simulink model "Speedmeter_harness"  (R2019b)
settings: Solver=FixedStepDiscrete  StartTime=0  StopTime=0.58999999999999997  FixedStep=0.01  RelTol=1e-3
undefined symbols (not defined in the file): Const16_0, Const16_2, Const16_210, Const16_340, Const16_350, Const16_4, Const8_0, Const8_1, Const8_2, Const8_4, ConstFL_00879, ConstFL_01, ConstFL_03516, ConstFL_1_6093, sigbuilder_block, STEP_TIME
libraries: simulink x2
(part 2 of 2)

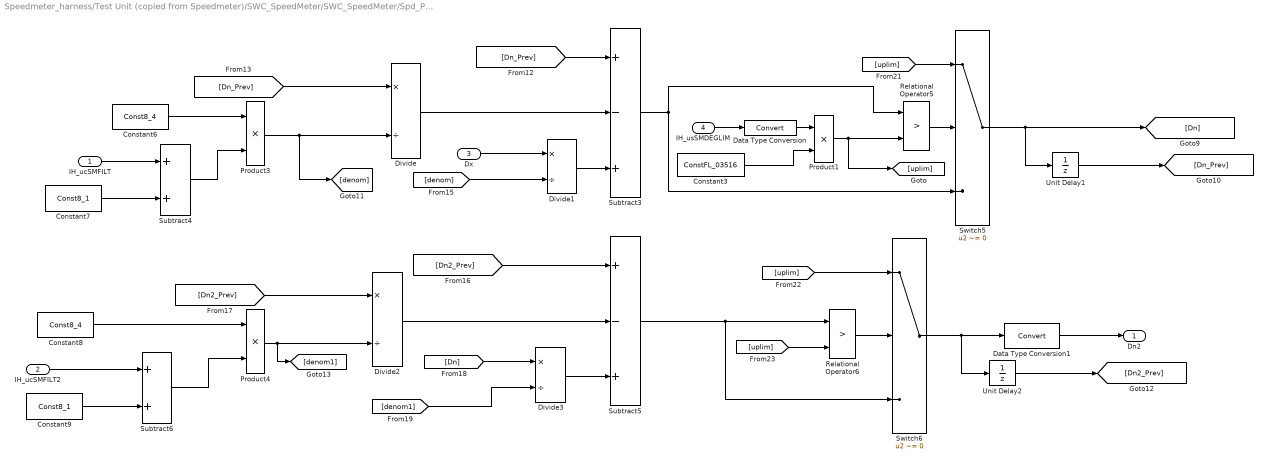
== system Speedmeter_harness/Test Unit (copied from Speedmeter)/SWC_SpeedMeter/SWC_SpeedMeter/Spd_Pointer/Filter ==
  IH_ucSMFILT : Inport  OutMin=0  OutMax=7  OutDataTypeStr=fixdt(0,8,1,0)  SampleTime=STEP_TIME
  IH_ucSMFILT2 : Inport  Port=2  OutMin=0  OutMax=7  OutDataTypeStr=fixdt(0,8,1,0)  SampleTime=STEP_TIME
  Dx : Inport  Port=3  SampleTime=STEP_TIME
  IH_usSMDEGLIM : Inport  Port=4  OutMin=0  OutMax=1023  SampleTime=STEP_TIME
  Constant3 : Constant  Value=ConstFL_03516  OutDataTypeStr=fixdt(0,32,0.0001,0)  SampleTime=STEP_TIME
  Constant6 : Constant  Value=Const8_4  SampleTime=STEP_TIME
  Constant7 : Constant  Value=Const8_1  OutDataTypeStr=uint8  SampleTime=STEP_TIME
  Constant8 : Constant  Value=Const8_4  SampleTime=STEP_TIME
  Constant9 : Constant  Value=Const8_1  SampleTime=STEP_TIME
  Data Type Conversion : DataTypeConversion
  Data Type Conversion1 : DataTypeConversion  SaturateOnIntegerOverflow=on
  Divide{,1..3} (4 alike) : Product  Inputs=*/  OutDataTypeStr=Inherit: Inherit via back propagation  InputSameDT=on
  Product1 : Product  OutDataTypeStr=fixdt(1,32,0.0001,0)  InputSameDT=on
  Product3 : Product  OutDataTypeStr=fixdt(1,32,0.0001,0)  InputSameDT=on
  Product4 : Product  OutDataTypeStr=fixdt(1,32,0.0001,0)  InputSameDT=on
  Relational Operator5 : RelationalOperator  Operator=>  OutDataTypeStr=boolean  RndMeth=Simplest  InputSameDT=on
  Relational Operator6 : RelationalOperator  Operator=>  OutDataTypeStr=boolean  RndMeth=Simplest  InputSameDT=on
  Subtract3 : Sum  Inputs=+-+  InputSameDT=on
  Subtract4 : Sum  InputSameDT=on
  Subtract5 : Sum  Inputs=+-+  OutDataTypeStr=Inherit: Inherit via back propagation  InputSameDT=on
  Subtract6 : Sum  InputSameDT=on
  Switch5 : Switch  Criteria=u2 ~= 0  InputSameDT=on
  Switch6 : Switch  Criteria=u2 ~= 0  OutDataTypeStr=Inherit: Inherit via back propagation  InputSameDT=on
  Unit Delay1 : UnitDelay  SampleTime=-1  HasFrameUpgradeWarning=on
  Unit Delay2 : UnitDelay  SampleTime=-1  HasFrameUpgradeWarning=on
  Dn2 : Outport  SampleTime=STEP_TIME  VectorParamsAs1DForOutWhenUnconnected=off
  wires:
  Divide1/1 -> Subtract3/3
  IH_ucSMFILT/1 -> Subtract4/1
  Subtract5/1 -> Switch6/3, Relational Operator6/1
  Constant9/1 -> Subtract6/2
  Subtract6/1 -> Product4/2
  [uplim] -> Switch5/1
  Divide3/1 -> Subtract5/3
  Switch6/1 -> Unit Delay2/1, Data Type Conversion1/1
  [Dn2_Prev] -> Divide2/1
  [Dn_Prev] -> Divide/1
  Unit Delay2/1 -> [Dn2_Prev]
  [uplim] -> Switch6/1
  [denom] -> Divide1/2
  Divide/1 -> Subtract3/2
  Data Type Conversion/1 -> Product1/1
  [Dn_Prev] -> Subtract3/1
  Relational Operator6/1 -> Switch6/2
  Constant7/1 -> Subtract4/2
  IH_usSMDEGLIM/1 -> Data Type Conversion/1
  Relational Operator5/1 -> Switch5/2
  Dx/1 -> Divide1/1
  Constant3/1 -> Product1/2
  IH_ucSMFILT2/1 -> Subtract6/1
  Constant8/1 -> Product4/1
  [denom1] -> Divide3/2
  [Dn] -> Divide3/1
  Product4/1 -> Divide2/2, [denom1]
  Product1/1 -> Relational Operator5/2, [uplim]
  Unit Delay1/1 -> [Dn_Prev]
  Switch5/1 -> [Dn], Unit Delay1/1
  Product3/1 -> [denom], Divide/2
  Subtract3/1 -> Switch5/3, Relational Operator5/1
  Subtract4/1 -> Product3/2
  [Dn2_Prev] -> Subtract5/1
  [uplim] -> Relational Operator6/2
  Constant6/1 -> Product3/1
  Divide2/1 -> Subtract5/2
  Data Type Conversion1/1 -> Dn2/1

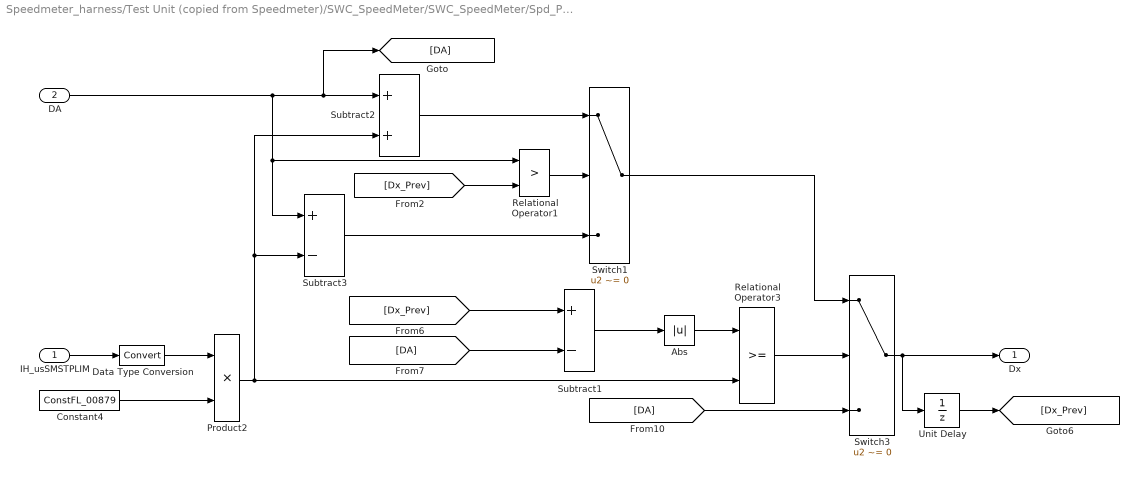
== system Speedmeter_harness/Test Unit (copied from Speedmeter)/SWC_SpeedMeter/SWC_SpeedMeter/Spd_Pointer/InputLimitProccess ==
  IH_usSMSTPLIM : Inport  SampleTime=STEP_TIME
  DA : Inport  Port=2  SampleTime=STEP_TIME
  Abs : Abs  OutDataTypeStr=fixdt(1,32,0.0001,0)
  Constant4 : Constant  Value=ConstFL_00879  OutDataTypeStr=fixdt(0,32,0.0001,0)  SampleTime=STEP_TIME
  Data Type Conversion : DataTypeConversion
  Product2 : Product  OutDataTypeStr=Inherit: Inherit via back propagation  InputSameDT=on
  Relational Operator1 : RelationalOperator  Operator=>  OutDataTypeStr=boolean  RndMeth=Simplest  InputSameDT=on
  Relational Operator3 : RelationalOperator  OutDataTypeStr=boolean  RndMeth=Simplest  InputSameDT=on
  Subtract1 : Sum  Inputs=+-  InputSameDT=on
  Subtract2 : Sum  InputSameDT=on
  Subtract3 : Sum  Inputs=+-  InputSameDT=on
  Switch1 : Switch  Criteria=u2 ~= 0  OutDataTypeStr=Inherit: Inherit via back propagation  InputSameDT=on
  Switch3 : Switch  Criteria=u2 ~= 0  OutDataTypeStr=Inherit: Inherit via back propagation  InputSameDT=on
  Unit Delay : UnitDelay  SampleTime=-1  HasFrameUpgradeWarning=on
  Dx : Outport  SampleTime=STEP_TIME  VectorParamsAs1DForOutWhenUnconnected=off
  wires:
  Unit Delay/1 -> [Dx_Prev]
  DA/1 -> Subtract2/1, [DA], Relational Operator1/1, Subtract3/1
  [Dx_Prev] -> Subtract1/1
  Product2/1 -> Subtract3/2, Subtract2/2, Relational Operator3/2
  Data Type Conversion/1 -> Product2/1
  IH_usSMSTPLIM/1 -> Data Type Conversion/1
  Abs/1 -> Relational Operator3/1
  [DA] -> Switch3/3
  Switch3/1 -> Unit Delay/1, Dx/1
  Subtract1/1 -> Abs/1
  Subtract2/1 -> Switch1/1
  [DA] -> Subtract1/2
  Relational Operator3/1 -> Switch3/2
  Relational Operator1/1 -> Switch1/2
  Switch1/1 -> Switch3/1
  Subtract3/1 -> Switch1/3
  [Dx_Prev] -> Relational Operator1/2
  Constant4/1 -> Product2/2

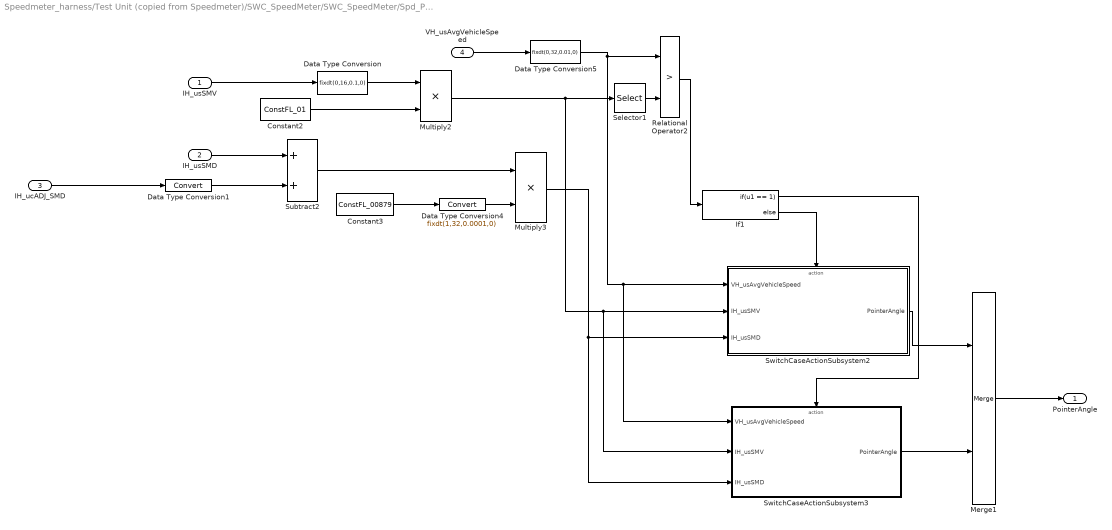
== system Speedmeter_harness/Test Unit (copied from Speedmeter)/SWC_SpeedMeter/SWC_SpeedMeter/Spd_Pointer/PointerAngleCalculation ==
  IH_usSMV : Inport  SampleTime=STEP_TIME
  IH_usSMD : Inport  Port=2  SampleTime=STEP_TIME
  IH_ucADJ_SMD : Inport  Port=3  SampleTime=STEP_TIME
  VH_usAvgVehicleSpeed : Inport  Port=4  SampleTime=STEP_TIME
  Constant2 : Constant  Value=ConstFL_01  SampleTime=STEP_TIME
  Constant3 : Constant  Value=ConstFL_00879  SampleTime=STEP_TIME
  Data Type Conversion : DataTypeConversion  OutDataTypeStr=fixdt(0,16,0.1,0)
  Data Type Conversion1 : DataTypeConversion
  Data Type Conversion4 : DataTypeConversion  OutDataTypeStr=fixdt(1,32,0.0001,0)
  Data Type Conversion5 : DataTypeConversion  OutDataTypeStr=fixdt(0,32,0.01,0)
  If1 : If  IfExpression=u1 == 1
  Merge1 : Merge  InitialOutput=0
  Multiply2 : Product  OutDataTypeStr=fixdt(0,32,0.01,0)  InputSameDT=on
  Multiply3 : Product  InputSameDT=on  OutDataTypeStr=Inherit: Same as first input
  Relational Operator2 : RelationalOperator  Operator=>  OutDataTypeStr=boolean  RndMeth=Simplest
  Selector1 : Selector  IndexMode=Zero-based  InputPortWidth=13  IndexOptions=Index vector (dialog)  Indices=[12]  OutputSizes=1
  Subtract2 : Sum  OutDataTypeStr=Inherit: Inherit via back propagation  InputSameDT=on
  SwitchCaseActionSubsystem2 : Subsystem  TreatAsAtomicUnit=on
  SwitchCaseActionSubsystem3 : Subsystem  TreatAsAtomicUnit=on
  PointerAngle : Outport  SampleTime=STEP_TIME  VectorParamsAs1DForOutWhenUnconnected=off
  wires:
  Data Type Conversion1/1 -> Subtract2/2
  Multiply3/1 -> SwitchCaseActionSubsystem3/3(IH_usSMD), SwitchCaseActionSubsystem2/3(IH_usSMD)
  IH_usSMV/1 -> Data Type Conversion/1
  VH_usAvgVehicleSpeed/1 -> Data Type Conversion5/1
  Constant3/1 -> Data Type Conversion4/1
  SwitchCaseActionSubsystem2/1(PointerAngle) -> Merge1/1
  Data Type Conversion/1 -> Multiply2/1
  Data Type Conversion5/1 -> Relational Operator2/1, SwitchCaseActionSubsystem3/1(VH_usAvgVehicleSpeed), SwitchCaseActionSubsystem2/1(VH_usAvgVehicleSpeed)
  Subtract2/1 -> Multiply3/1
  Relational Operator2/1 -> If1/1
  Merge1/1 -> PointerAngle/1
  Multiply2/1 -> SwitchCaseActionSubsystem3/2(IH_usSMV), SwitchCaseActionSubsystem2/2(IH_usSMV), Selector1/1
  Data Type Conversion4/1 -> Multiply3/2
  SwitchCaseActionSubsystem3/1(PointerAngle) -> Merge1/2
  If1/2 -> SwitchCaseActionSubsystem2/Action
  IH_usSMD/1 -> Subtract2/1
  If1/1 -> SwitchCaseActionSubsystem3/Action
  IH_ucADJ_SMD/1 -> Data Type Conversion1/1
  Selector1/1 -> Relational Operator2/2
  Constant2/1 -> Multiply2/2

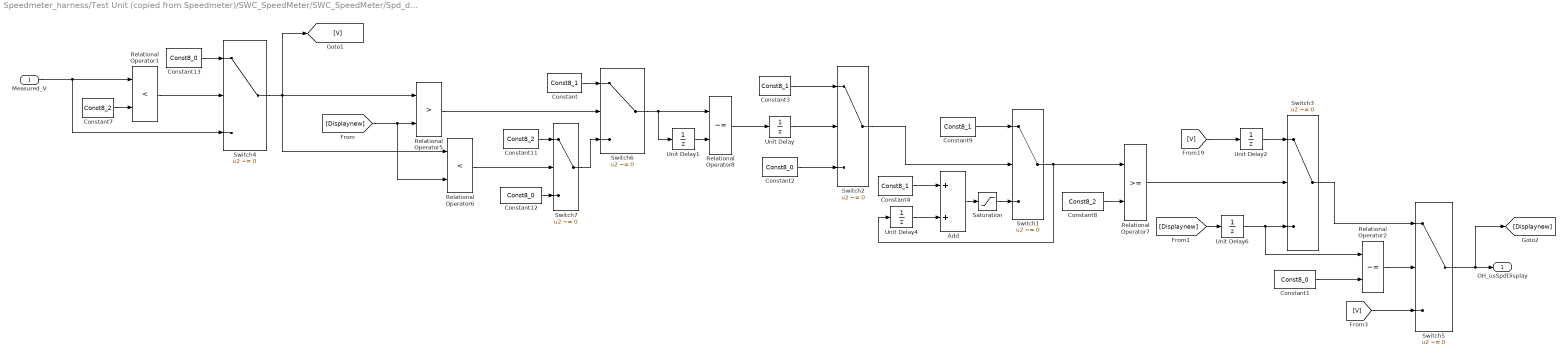
== system Speedmeter_harness/Test Unit (copied from Speedmeter)/SWC_SpeedMeter/SWC_SpeedMeter/Spd_disp/Displayfilter ==
  Measured_V : Inport  OutDataTypeStr=fixdt(0,16,1,0)
  Add : Sum  InputSameDT=on
  Constant{,3..4,9} (4 alike) : Constant  Value=Const8_1
  Constant1 : Constant  Value=Const8_0  OutDataTypeStr=Inherit: Inherit via back propagation
  Constant11 : Constant  Value=Const8_2
  Constant12 : Constant  Value=Const8_0
  Constant13 : Constant  Value=Const8_0  OutDataTypeStr=Inherit: Inherit via back propagation
  Constant2 : Constant  Value=Const8_0
  Constant7 : Constant  Value=Const8_2  OutDataTypeStr=Inherit: Inherit via back propagation
  Constant8 : Constant  Value=Const8_2
  Relational Operator1 : RelationalOperator  Operator=<  OutDataTypeStr=boolean  RndMeth=Simplest  InputSameDT=on
  Relational Operator2 : RelationalOperator  Operator=~=  OutDataTypeStr=boolean  RndMeth=Simplest  InputSameDT=on
  Relational Operator5 : RelationalOperator  Operator=>  OutDataTypeStr=boolean  RndMeth=Simplest  InputSameDT=on
  Relational Operator6 : RelationalOperator  Operator=<  OutDataTypeStr=boolean  RndMeth=Simplest  InputSameDT=on
  Relational Operator7 : RelationalOperator  OutDataTypeStr=boolean  RndMeth=Simplest  InputSameDT=on
  Relational Operator8 : RelationalOperator  Operator=~=  OutDataTypeStr=boolean  RndMeth=Simplest  InputSameDT=on
  Saturation : Saturate  UpperLimit=3  LowerLimit=1  OutDataTypeStr=uint8
  Switch1 : Switch  Criteria=u2 ~= 0  Threshold=2  InputSameDT=on
  Switch2 : Switch  Criteria=u2 ~= 0  Threshold=2  InputSameDT=on
  Switch3 : Switch  Criteria=u2 ~= 0  OutDataTypeStr=Inherit: Inherit via back propagation  InputSameDT=on
  Switch{4..7} (4 alike) : Switch  Criteria=u2 ~= 0  InputSameDT=on
  Unit Delay{,1..2,4,6} (5 alike) : UnitDelay  SampleTime=-1  HasFrameUpgradeWarning=on
  OH_usSpdDisplay : Outport  OutDataTypeStr=fixdt(0,16,1,0)  VectorParamsAs1DForOutWhenUnconnected=off
  wires:
  Switch2/1 -> Switch1/2
  Switch5/1 -> OH_usSpdDisplay/1, [Displaynew]
  Relational Operator8/1 -> Unit Delay/1
  Unit Delay4/1 -> Add/2
  Relational Operator2/1 -> Switch5/2
  Switch4/1 -> Relational Operator6/1, Relational Operator5/1, [V]
  Constant8/1 -> Relational Operator7/2
  [Displaynew] -> Relational Operator6/2, Relational Operator5/2
  Switch1/1 -> Unit Delay4/1, Relational Operator7/1
  Relational Operator1/1 -> Switch4/2
  Unit Delay6/1 -> Switch3/3, Relational Operator2/1
  Constant4/1 -> Add/1
  Unit Delay1/1 -> Relational Operator8/2
  Switch6/1 -> Relational Operator8/1, Unit Delay1/1
  Constant2/1 -> Switch2/3
  Add/1 -> Saturation/1
  Unit Delay/1 -> Switch2/2
  Switch3/1 -> Switch5/1
  Constant11/1 -> Switch7/1
  Constant3/1 -> Switch2/1
  Measured_V/1 -> Relational Operator1/1, Switch4/3
  Constant12/1 -> Switch7/3
  [Displaynew] -> Unit Delay6/1
  Constant/1 -> Switch6/1
  Switch7/1 -> Switch6/3
  Constant9/1 -> Switch1/1
  Constant7/1 -> Relational Operator1/2
  Saturation/1 -> Switch1/3
  Unit Delay2/1 -> Switch3/1
  Constant1/1 -> Relational Operator2/2
  [V] -> Switch5/3
  Relational Operator5/1 -> Switch6/2
  Relational Operator6/1 -> Switch7/2
  Relational Operator7/1 -> Switch3/2
  Constant13/1 -> Switch4/1
  [V] -> Unit Delay2/1

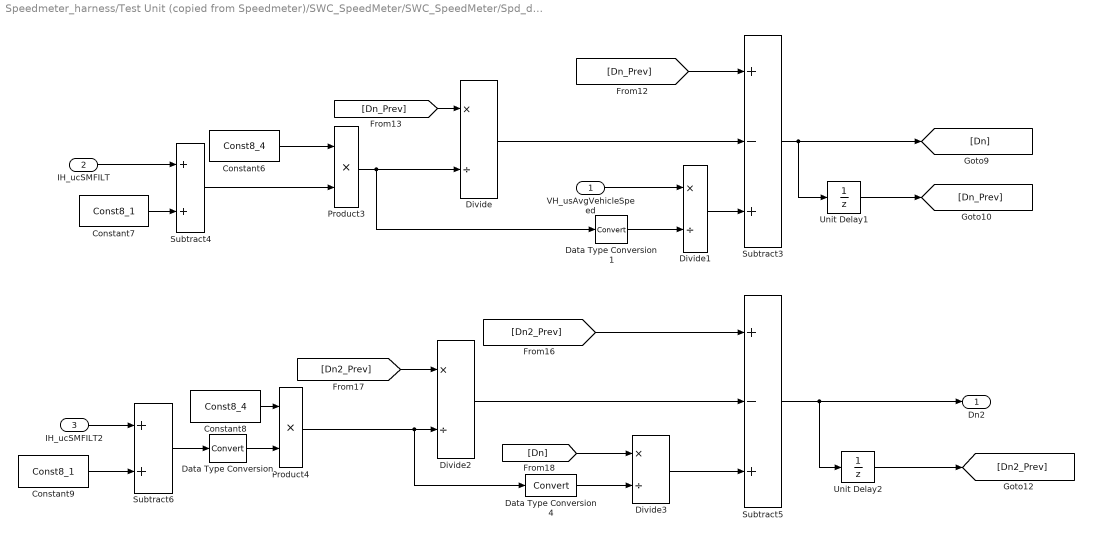
== system Speedmeter_harness/Test Unit (copied from Speedmeter)/SWC_SpeedMeter/SWC_SpeedMeter/Spd_disp/FilteringProcess ==
  VH_usAvgVehicleSpeed : Inport  SampleTime=STEP_TIME
  IH_ucSMFILT : Inport  Port=2  OutDataTypeStr=fixdt(0,8,1,0)  SampleTime=STEP_TIME
  IH_ucSMFILT2 : Inport  Port=3  OutDataTypeStr=fixdt(0,8,1,0)  SampleTime=STEP_TIME
  Constant6 : Constant  Value=Const8_4  SampleTime=STEP_TIME
  Constant7 : Constant  Value=Const8_1  SampleTime=STEP_TIME
  Constant8 : Constant  Value=Const8_4  SampleTime=STEP_TIME
  Constant9 : Constant  Value=Const8_1  SampleTime=STEP_TIME
  Data Type Conversion : DataTypeConversion
  Data Type Conversion1 : DataTypeConversion
  Data Type Conversion4 : DataTypeConversion
  Divide{,1..3} (4 alike) : Product  Inputs=*/  OutDataTypeStr=fixdt(0,16,0.1,0)  InputSameDT=on
  Product3 : Product  OutDataTypeStr=Inherit: Inherit via back propagation  InputSameDT=on
  Product4 : Product  OutDataTypeStr=Inherit: Inherit via back propagation  InputSameDT=on
  Subtract3 : Sum  Inputs=+-+  InputSameDT=on
  Subtract4 : Sum  InputSameDT=on
  Subtract5 : Sum  Inputs=+-+  InputSameDT=on
  Subtract6 : Sum  OutDataTypeStr=uint16  InputSameDT=on
  Unit Delay1 : UnitDelay  SampleTime=-1  HasFrameUpgradeWarning=on
  Unit Delay2 : UnitDelay  SampleTime=-1  HasFrameUpgradeWarning=on
  Dn2 : Outport  SampleTime=STEP_TIME  VectorParamsAs1DForOutWhenUnconnected=off
  wires:
  Unit Delay2/1 -> [Dn2_Prev]
  [Dn2_Prev] -> Subtract5/1
  Data Type Conversion4/1 -> Divide3/2
  Unit Delay1/1 -> [Dn_Prev]
  [Dn_Prev] -> Subtract3/1
  Data Type Conversion1/1 -> Divide1/2
  Data Type Conversion/1 -> Product4/2
  Constant9/1 -> Subtract6/2
  Divide1/1 -> Subtract3/3
  Constant8/1 -> Product4/1
  Divide/1 -> Subtract3/2
  Subtract3/1 -> [Dn], Unit Delay1/1
  Subtract6/1 -> Data Type Conversion/1
  VH_usAvgVehicleSpeed/1 -> Divide1/1
  [Dn_Prev] -> Divide/1
  IH_ucSMFILT2/1 -> Subtract6/1
  Constant7/1 -> Subtract4/2
  [Dn] -> Divide3/1
  Product4/1 -> Divide2/2, Data Type Conversion4/1
  [Dn2_Prev] -> Divide2/1
  Subtract4/1 -> Product3/2
  Product3/1 -> Divide/2, Data Type Conversion1/1
  Divide3/1 -> Subtract5/3
  Divide2/1 -> Subtract5/2
  Constant6/1 -> Product3/1
  IH_ucSMFILT/1 -> Subtract4/1
  Subtract5/1 -> Unit Delay2/1, Dn2/1

== system Speedmeter_harness/Test Unit (copied from Speedmeter)/SWC_SpeedMeter/SWC_SpeedMeter/Spd_disp/UnitConversion ==
  OH_ucSetUnitSpeed : Inport  OutDataTypeStr=fixdt(0,8,1,0)  SampleTime=STEP_TIME
  Dn2 : Inport  Port=2  OutDataTypeStr=fixdt(0,16,0.1,0)  SampleTime=STEP_TIME
  Constant : Constant  Value=ConstFL_1_6093  SampleTime=STEP_TIME
  Constant1 : Constant  Value=Const8_1  SampleTime=STEP_TIME
  Constant10 : Constant  Value=Const16_340  SampleTime=STEP_TIME
  Constant11 : Constant  Value=Const16_340  SampleTime=STEP_TIME
  Constant4 : Constant  Value=Const16_210  OutDataTypeStr=Inherit: Inherit via back propagation  SampleTime=STEP_TIME
  Constant5 : Constant  Value=Const16_210  OutDataTypeStr=Inherit: Inherit via back propagation  SampleTime=STEP_TIME
  Data Type Conversion1 : DataTypeConversion
  Data Type Conversion2 : DataTypeConversion  OutDataTypeStr=fixdt(0,32,0.0001,0)
  Data Type Conversion3 : DataTypeConversion
  Data Type Conversion4 : DataTypeConversion
  Divide6 : Product  Inputs=*/  OutDataTypeStr=fixdt(0,16,0.01,0)  InputSameDT=on
  Relational Operator2 : RelationalOperator  Operator=>  OutDataTypeStr=boolean  RndMeth=Simplest  InputSameDT=on
  Relational Operator3 : RelationalOperator  Operator=>  OutDataTypeStr=boolean  RndMeth=Simplest  InputSameDT=on
  Relational Operator5 : RelationalOperator  Operator===  OutDataTypeStr=boolean  RndMeth=Simplest  InputSameDT=on
  Switch2 : Switch  Criteria=u2 ~= 0  OutDataTypeStr=Inherit: Inherit via back propagation  InputSameDT=on
  Switch3 : Switch  Criteria=u2 ~= 0  InputSameDT=on
  Switch5 : Switch  Criteria=u2 ~= 0  OutDataTypeStr=Inherit: Inherit via back propagation  InputSameDT=on
  Measured_V : Outport  OutDataTypeStr=fixdt(0,16,1,0)  SampleTime=STEP_TIME  VectorParamsAs1DForOutWhenUnconnected=off
  wires:
  Data Type Conversion4/1 -> Divide6/2
  Data Type Conversion3/1 -> Switch3/1
  Constant4/1 -> Relational Operator2/2
  Switch5/1 -> Measured_V/1
  Data Type Conversion2/1 -> Divide6/1
  Switch2/1 -> Switch5/1
  Switch3/1 -> Switch5/3
  Relational Operator5/1 -> Switch5/2
  Constant5/1 -> Switch2/1
  Divide6/1 -> Switch2/3, Relational Operator2/1
  Data Type Conversion1/1 -> Relational Operator3/2
  Constant11/1 -> Data Type Conversion3/1
  Relational Operator2/1 -> Switch2/2
  Relational Operator3/1 -> Switch3/2
  Constant/1 -> Data Type Conversion4/1
  Constant10/1 -> Data Type Conversion1/1
  Constant1/1 -> Relational Operator5/2
  Dn2/1 -> Data Type Conversion2/1, Switch3/3, Relational Operator3/1
  OH_ucSetUnitSpeed/1 -> Relational Operator5/1

== system Speedmeter_harness/Test Unit (copied from Speedmeter)/SWC_SpeedMeter/SWC_SpeedMeter/Spd_Pointer/PointerAngleCalculation/SwitchCaseActionSubsystem2 ==
  VH_usAvgVehicleSpeed : Inport  PortDimensions=1  SampleTime=STEP_TIME
  IH_usSMV : Inport  Port=2  OutMin=0  OutMax=4095  SampleTime=STEP_TIME
  IH_usSMD : Inport  Port=3  OutMin=0  OutMax=4095  SampleTime=STEP_TIME
  Action Port : ActionPort
  Lookup Table Dynamic : simulink/Lookup Tables/Lookup Table Dynamic  LookUpMeth=Interpolation-Use End Values  OutDataType=fixdt(0,16,0.1,0)  OutScaling=[]  OutDataTypeStr=Inherit: Inherit via back propagation  DoSatur=off
      settings: SourceProductName=Simulink
  PointerAngle : Outport  SampleTime=STEP_TIME  VectorParamsAs1DForOutWhenUnconnected=off
  wires:
  IH_usSMD/1 -> Lookup Table Dynamic/3
  Lookup Table Dynamic/1 -> PointerAngle/1
  IH_usSMV/1 -> Lookup Table Dynamic/2
  VH_usAvgVehicleSpeed/1 -> Lookup Table Dynamic/1

== system Speedmeter_harness/Test Unit (copied from Speedmeter)/SWC_SpeedMeter/SWC_SpeedMeter/Spd_Pointer/PointerAngleCalculation/SwitchCaseActionSubsystem3 ==
  VH_usAvgVehicleSpeed : Inport  SampleTime=STEP_TIME
  IH_usSMV : Inport  Port=2  OutMin=0  OutMax=4095  SampleTime=STEP_TIME
  IH_usSMD : Inport  Port=3  OutMin=0  OutMax=4095  SampleTime=STEP_TIME
  Action Port : ActionPort
  Divide : Product  Inputs=*/  OutDataTypeStr=Inherit: Inherit via back propagation  SaturateOnIntegerOverflow=on  InputSameDT=on
  Multiply3 : Product  OutDataTypeStr=Inherit: Inherit via back propagation  InputSameDT=on
  Selector : Selector  IndexMode=Zero-based  InputPortWidth=13  IndexOptions=Index vector (dialog)  Indices=[11]  OutputSizes=1
  Selector1 : Selector  IndexMode=Zero-based  InputPortWidth=13  IndexOptions=Index vector (dialog)  Indices=[12]  OutputSizes=1
  Selector2 : Selector  IndexMode=Zero-based  InputPortWidth=13  IndexOptions=Index vector (dialog)  Indices=[12]  OutputSizes=1
  Selector3 : Selector  IndexMode=Zero-based  InputPortWidth=13  IndexOptions=Index vector (dialog)  Indices=[11]  OutputSizes=1
  Subtract1 : Sum  Inputs=+-  OutDataTypeStr=Inherit: Inherit via back propagation  InputSameDT=on
  Subtract2 : Sum  Inputs=+-  InputSameDT=on  OutDataTypeStr=Inherit: Same as first input
  Subtract3 : Sum  Inputs=+-  OutDataTypeStr=Inherit: Inherit via back propagation  InputSameDT=on
  Subtract4 : Sum  OutDataTypeStr=Inherit: Inherit via back propagation  InputSameDT=on
  PointerAngle : Outport  SampleTime=STEP_TIME  VectorParamsAs1DForOutWhenUnconnected=off
  wires:
  Selector1/1 -> Subtract3/1
  Subtract3/1 -> Divide/2
  IH_usSMD/1 -> Selector2/1, Selector3/1
  IH_usSMV/1 -> Selector1/1, Selector/1
  Subtract2/1 -> Multiply3/1
  Divide/1 -> Multiply3/2
  Selector2/1 -> Subtract2/1
  Multiply3/1 -> Subtract4/1
  Selector/1 -> Subtract1/2, Subtract3/2
  Selector3/1 -> Subtract2/2, Subtract4/2
  Subtract1/1 -> Divide/1
  VH_usAvgVehicleSpeed/1 -> Subtract1/1
  Subtract4/1 -> PointerAngle/1

== stateflow chart Speedmeter_harness/Test Unit (copied from Speedmeter)/SWC_SpeedMeter/SWC_SpeedMeter/Spd_Common/HeapSort ==
  state K1  = HeapSort(InitPos, Len, N) [function]
    note: /*Perform Heapsort sorting for Key array K
        | Input Argument:
        | InitPos:Start index position for sorting
        | Len:	Len the of the values in array to be sorted
        | N:	Key array
        | PriOrderArr:	2-D array
        |
        | Output Argument:
        | K1= Sorted Key array;
        | HeapifyOut = Sorted 2-D array
        | Flag = Contains status of sorting algorithm
        | */
    (default) -> (junction 2826)
    (junction 2826) -> (junction 2827) [order 1] : [Len <= 1]
        | {Flag = FALSE;}
    (junction 2826) -> (junction 2828) [order 2]
    (junction 2827) -> (junction 2833)
    (junction 2828) -> (junction 2829) [order 1] : [Len > R_MD_AD2ARNDCARMAX]
    (junction 2828) -> (junction 2830) [order 2]
    (junction 2829) -> (junction 2831) : {Len = R_MD_AD2ARNDCARMAX;}
    (junction 2831) -> (junction 2830)
    (junction 2830) -> (junction 2832)
    (junction 2832) -> (junction 2833) [order 1] : [InitPos < 0 ]
        | {Flag=FALSE;}
    (junction 2832) -> (junction 2834) [order 2]
    (junction 2833) -> (junction 2835)
    (junction 2834) -> (junction 2835) [order 1] : [((InitPos + Len - 1) >= R_MD_AD2ARNDCARMAX)]
        | {Flag=FALSE;}
    (junction 2834) -> (junction 2837) [order 2] : {
        | LNode = Len -1+InitPos ;
        | RNode = InitPos;}
    (junction 2835) -> (junction 2839)
    (junction 2836) -> (junction 2837)
    (junction 2864) -> (junction 2836)
    (junction 2837) -> (junction 2838)
    (junction 2838) -> (junction 2839) [order 2] : {Flag=TRUE;}
    (junction 2838) -> (junction 2841) [order 1] : [RNode <LNode]
        | {
        | PNode = (((LNode-1 - RNode ) )/2) + RNode;
        | MNode = PNode;
        | }
    (junction 2839) -> (junction 2853)
    (junction 2840) -> (junction 2841)
    (junction 2841) -> (junction 2843) : {CLNode = (2*PNode + 1) - RNode;
        | CRNode = (2*PNode + 2) - RNode;}
    (junction 2861) -> (junction 2840)
    (junction 2843) -> (junction 2842) [order 1] : [N[PNode] <= N[CLNode]]
    (junction 2843) -> (junction 2844) [order 2] : {select_val = N[CLNode];
        | select_node = CLNode;}
    (junction 2842) -> (junction 2845) : {select_val = N[PNode];
        | select_node = PNode;}
    (junction 2845) -> (junction 2844)
    (junction 2844) -> (junction 2846)
    (junction 2846) -> (junction 2847) [order 1] : [(CRNode <= LNode) ]
    (junction 2847) -> (junction 2848) [order 1] : [(select_val > N[CRNode])]
    (junction 2846) -> (junction 2849) [order 2] : {CRNode=0;}
    (junction 2847) -> (junction 2850) [order 2]
    (junction 2848) -> (junction 2851) : {select_val = N[CRNode];
        | select_node = CRNode;}
    (junction 2850) -> (junction 2849)
    (junction 2851) -> (junction 2850)
    (junction 2849) -> (junction 2854)
    (junction 2854) -> (junction 2855) [order 2]
    (junction 2855) -> (junction 2852) [order 2]
    (junction 2852) -> (junction 2853) [order 2] : {Flag=FALSE;}
    (junction 2854) -> (junction 2856) [order 1] : [N[select_node]==N[PNode]]
        | {MNode--;
        | PNode = MNode;}
    (junction 2855) -> (junction 2857) [order 1] : [N[select_node]==N[CLNode]]
        | {work_val = N[PNode];
        | N[PNode] = N[CLNode];
        | N[CLNode] = work_val;
        | PNode = CLNode;
        | }
    (junction 2852) -> (junction 2858) [order 1] : [CRNode>=2 && N[select_node]==N[CRNode]]
        | {work_val = N[PNode];
        | N[PNode] = N[CRNode];
        | N[CRNode] = work_val;
        | PNode = CRNode;
        | }
    (junction 2853) -> (junction 2866) : {  K1[0]=N[0];
        | K1[1]=N[1];
        | K1[2]=N[2];
        | K1[3]=N[3];
        | K1[4]=N[4];
        | K1[5]=N[5];
        | K1[6]=N[6];
        | K1[7]=N[7];
        | K1[8]=N[8];
        | K1[9]=N[9];
        | K1[10]=N[10];
        | K1[11]=N[11];
        | K1[12]=N[12];
        | K1[13]=N[13];
        | K1[14]=N[14];
        | K1[15]=N[15];}
    (junction 2856) -> (junction 2857)
    (junction 2858) -> (junction 2857)
    (junction 2857) -> (junction 2860) : {work_CLNode = (2*PNode + 1) - RNode;
        | }
    (junction 2860) -> (junction 2859) [order 1] : [work_CLNode > LNode]
    (junction 2859) -> (junction 2863) : {MNode--;
        | PNode = MNode;}
    (junction 2860) -> (junction 2862) [order 2]
    (junction 2862) -> (junction 2861) [order 2]
    (junction 2863) -> (junction 2862)
    (junction 2862) -> (junction 2865) [order 1] : [MNode < RNode]
    (junction 2865) -> (junction 2864) : {RNode++;}
  (default) -> (junction 1643) : {
      | K1Arr = yLineArr; /*Create array K1 with yline values*/
      | K = HeapSort(0, 16, K1Arr);/* Sort K1 using Heapsort*/
      | }
  data: InitPos function_input uint8; Len function_input uint8 size=1; N function_input fixdt(0,16,0.01,0) size=16; K1 function_output fixdt(0,16,0.01,0) size=16; FALSE constant boolean =0; TRUE constant boolean =1; CLNode local int8; CRNode local int8; LNode local int8; MNode local int8; PNode local int8; RNode local int8; work_val local fixdt(0,16,0.01,0); select_node local int8; select_val local fixdt(0,16,0.01,0); R_MD_AD2ARNDCARMAX constant uint8 =16; yLineArr input fixdt(0,16,0.01,0) size=16; work_CLNode local int8; Flag local int8; K output fixdt(0,16,0.01,0) size=16; K1Arr local fixdt(0,16,0.01,0) size=16
  data InitPos settings: description=$TL$ type=UInt8; $TL$
  data Len settings: description=$TL$ type=UInt8; $TL$
  data N settings: description=$TL$ type=UInt16; $TL$
  data K1 settings: description=$TL$ type=UInt16; $TL$
  data FALSE settings: description=$TL$ type=UInt8; $TL$
  data TRUE settings: description=$TL$ type=UInt8; $TL$
  data CLNode settings: description=$TL$ type=UInt16; $TL$
  data CRNode settings: description=$TL$ type=UInt16; $TL$
  data LNode settings: description=$TL$ type=UInt16; $TL$
  data MNode settings: description=$TL$ type=Int8; $TL$
  data PNode settings: description=$TL$ type=UInt16; $TL$
  data RNode settings: description=$TL$ type=UInt8; $TL$
  data work_val settings: description=$TL$ type=UInt16; $TL$
  data select_node settings: description=$TL$ type=UInt8; $TL$
  data select_val settings: description=$TL$ type=UInt16; $TL$
  data R_MD_AD2ARNDCARMAX settings: description=$TL$ type=UInt8; $TL$
  data yLineArr settings: description=$TL$ type=UInt16; $TL$
  data work_CLNode settings: description=$TL$ type=UInt16; $TL$
  data K settings: description=$TL$ type=UInt16; $TL$
